simulink model "final_2017"  (R2017b)
settings: Solver=FixedStepAuto  StartTime=0.0  StopTime=inf  FixedStep=0.01  RelTol=1e-3  EnableMultiTasking=on
libraries: arduinolib x12, simulink x3
settings Model: ExtModeTrigDuration=2  Creator=Sina  LastModifiedBy=sina_
settings DataIOCC: ReturnWorkspaceOutputs=on
settings OptimizationCC: EnhancedBackFolding=on  PassReuseOutputArgsAs=Individual arguments  ZeroExternalMemoryAtStartup=off  ZeroInternalMemoryAtStartup=off  MaxStackSize=64  OptimizeBlockOrder=speed  DifferentSizesBufferReuse=on
settings DebuggingCC: ParameterTunabilityLossMsg=error  UnconnectedInputMsg=none  UnconnectedOutputMsg=none  UnconnectedLineMsg=none  SFMachineParentedDataDiag=error
settings HardwareCC: ProdBitPerInt=16  ProdBitPerPointer=16  ProdBitPerSizeT=16  ProdBitPerPtrDiffT=16  ProdLargestAtomicFloat=None  ProdWordSize=8  ProdHWDeviceType=Atmel->AVR
settings SFSimCC: SimUseLocalCustomCode=on  MATLABDynamicMemAlloc=off
settings RTWCC: SystemTargetFile=ert.tlc  HardwareBoard=Arduino Uno  TLCOptions=-aInlineSetEventsForThisBaseRateFcn=TLC_FALSE -aSuppressMultiTaskScheduler=TLC_FALSE -aRateBasedStepFcn=1  TemplateMakefile=ert_default_tmf  RTWUseLocalCustomCode=on  Toolchain=Arduino AVR  BuildConfiguration=Faster Runs
settings CodeAppCC: ForceParamTrailComments=on  IgnoreCustomStorageClasses=off  OperatorAnnotations=on  SimulinkDataObjDesc=on  SFDataObjDesc=on  InsertBlockDesc=on
settings ERTTargetCC: SupportContinuousTime=on  SupportVariableSizeSignals=on  ExtModeTransport=3  ExtModeStaticAlloc=on  ExtModeStaticAllocSize=250  ExtModeMexFile=ext_xcp  ExtModeIntrfLevel=Level2 - Open

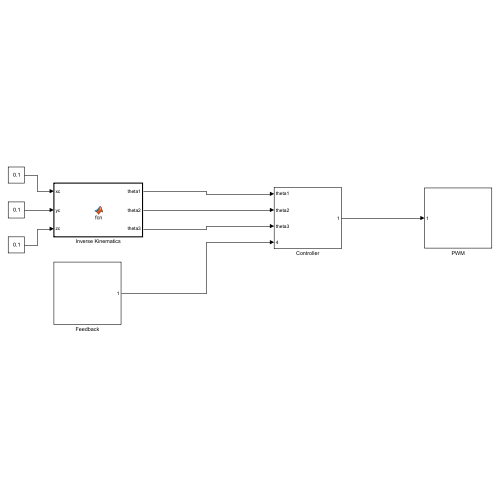
[thumbnail: Simulink's stored preview of the top-level diagram]
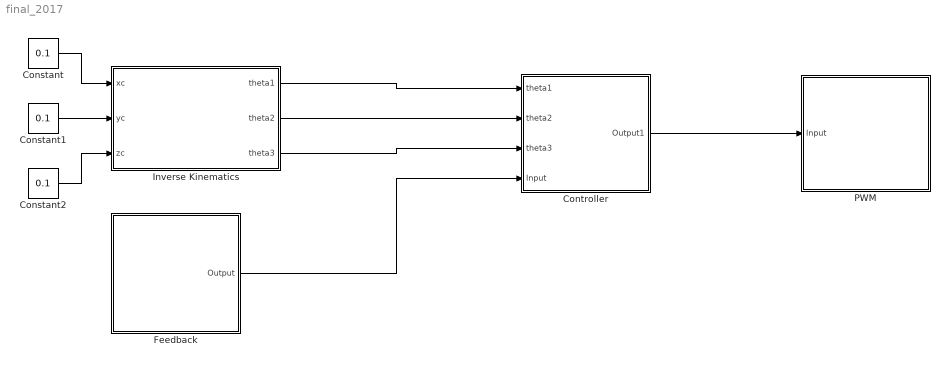
== system final_2017 ==
  Constant : Constant  Value=0.1
  Constant1 : Constant  Value=0.1
  Constant2 : Constant  Value=0.1
  Controller : Subsystem
  Feedback : Subsystem
  Inverse Kinematics : MATLAB Function  TreatAsAtomicUnit=on
  PWM : Subsystem
  wires:
  Feedback/1(Output) -> Controller/4(Input)
  Constant1/1 -> Inverse Kinematics/2(yc)
  Controller/1(Output1) -> PWM/1(Input)
  Constant/1 -> Inverse Kinematics/1(xc)
  Constant2/1 -> Inverse Kinematics/3(zc)
  Inverse Kinematics/1(theta1) -> Controller/1(theta1)
  Inverse Kinematics/2(theta2) -> Controller/2(theta2)
  Inverse Kinematics/3(theta3) -> Controller/3(theta3)

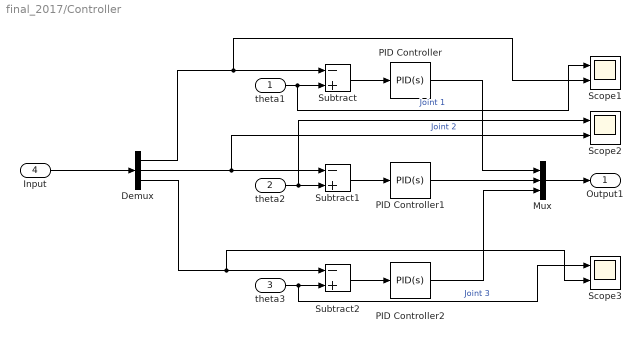
== system final_2017/Controller ==
  theta1 : Inport
  theta2 : Inport  Port=2
  theta3 : Inport  Port=3
  Input : Inport  Port=4
  Demux : Demux  Outputs=3
  Mux : Mux  Inputs=3
  PID Controller : simulink/Continuous/PID Controller  Controller=PID  Form=Parallel  TimeDomain=Continuous-time  SampleTime=-1  IntegratorMethod=Forward Euler  ControllerParametersSource=internal  P=5  I=2  D=1  N=100  UseFilter=on  TunerSelectOption=Transfer Function Based (PID Tuner App)  InitialConditionSource=internal  InitialConditionForIntegrator=0  InitialConditionForFilter=0  DifferentiatorICPrevScaledInput=0  ExternalReset=none  TrackingMode=off  Kt=1  LimitOutput=off  UpperSaturationLimit=inf  LowerSaturationLimit=-inf  LinearizeAsGain=on  AntiWindupMode=none  Kb=1  POutMin=[]  POutMax=[]  IOutMin=[]  IOutMax=[]  DOutMin=[]  DOutMax=[]  NOutMin=[]  NOutMax=[]  SumOutMin=[]  SumOutMax=[]  SaturationOutMin=[]  SaturationOutMax=[]  PParamMin=[]  PParamMax=[]  IParamMin=[]  IParamMax=[]  DParamMin=[]  DParamMax=[]  NParamMin=[]  NParamMax=[]  KbParamMin=[]  KbParamMax=[]  KtParamMin=[]  KtParamMax=[]  KbOutMin=[]  KbOutMax=[]  KtOutMin=[]  KtOutMax=[]  IntegratorOutMin=[]  IntegratorOutMax=[]  FilterOutMin=[]  FilterOutMax=[]  SumI1OutMin=[]  SumI1OutMax=[]  SumI2OutMin=[]  SumI2OutMax=[]  SumI3OutMin=[]  SumI3OutMax=[]  SumDOutMin=[]  SumDOutMax=[]  DifferentiatorOutMin=[]  DifferentiatorOutMax=[]  FilterDiffOutCoefMin=[]  FilterDiffOutCoefMax=[]  ReciprocalOutMin=[]  ReciprocalOutMax=[]  SumDenOutMin=[]  SumDenOutMax=[]  SumNumOutMin=[]  SumNumOutMax=[]  DivideOutMin=[]  DivideOutMax=[]  IntegratorContinuousStateAttributes=''  IntegratorStateMustResolveToSignalObject=off  IntegratorRTWStateStorageClass=Auto  FilterContinuousStateAttributes=''  FilterStateMustResolveToSignalObject=off  FilterRTWStateStorageClass=Auto  InitialConditionSetting=State (most efficient)
  PID Controller1 : simulink/Continuous/PID Controller  Controller=PID  Form=Parallel  TimeDomain=Continuous-time  SampleTime=-1  IntegratorMethod=Forward Euler  ControllerParametersSource=internal  P=5  I=2  D=1  N=100  UseFilter=on  TunerSelectOption=Transfer Function Based (PID Tuner App)  InitialConditionSource=internal  InitialConditionForIntegrator=0  InitialConditionForFilter=0  DifferentiatorICPrevScaledInput=0  ExternalReset=none  TrackingMode=off  Kt=1  LimitOutput=off  UpperSaturationLimit=inf  LowerSaturationLimit=-inf  LinearizeAsGain=on  AntiWindupMode=none  Kb=1  POutMin=[]  POutMax=[]  IOutMin=[]  IOutMax=[]  DOutMin=[]  DOutMax=[]  NOutMin=[]  NOutMax=[]  SumOutMin=[]  SumOutMax=[]  SaturationOutMin=[]  SaturationOutMax=[]  PParamMin=[]  PParamMax=[]  IParamMin=[]  IParamMax=[]  DParamMin=[]  DParamMax=[]  NParamMin=[]  NParamMax=[]  KbParamMin=[]  KbParamMax=[]  KtParamMin=[]  KtParamMax=[]  KbOutMin=[]  KbOutMax=[]  KtOutMin=[]  KtOutMax=[]  IntegratorOutMin=[]  IntegratorOutMax=[]  FilterOutMin=[]  FilterOutMax=[]  SumI1OutMin=[]  SumI1OutMax=[]  SumI2OutMin=[]  SumI2OutMax=[]  SumI3OutMin=[]  SumI3OutMax=[]  SumDOutMin=[]  SumDOutMax=[]  DifferentiatorOutMin=[]  DifferentiatorOutMax=[]  FilterDiffOutCoefMin=[]  FilterDiffOutCoefMax=[]  ReciprocalOutMin=[]  ReciprocalOutMax=[]  SumDenOutMin=[]  SumDenOutMax=[]  SumNumOutMin=[]  SumNumOutMax=[]  DivideOutMin=[]  DivideOutMax=[]  IntegratorContinuousStateAttributes=''  IntegratorStateMustResolveToSignalObject=off  IntegratorRTWStateStorageClass=Auto  FilterContinuousStateAttributes=''  FilterStateMustResolveToSignalObject=off  FilterRTWStateStorageClass=Auto  InitialConditionSetting=State (most efficient)
  PID Controller2 : simulink/Continuous/PID Controller  Controller=PID  Form=Parallel  TimeDomain=Continuous-time  SampleTime=-1  IntegratorMethod=Forward Euler  ControllerParametersSource=internal  P=5  I=2  D=1  N=100  UseFilter=on  TunerSelectOption=Transfer Function Based (PID Tuner App)  InitialConditionSource=internal  InitialConditionForIntegrator=0  InitialConditionForFilter=0  DifferentiatorICPrevScaledInput=0  ExternalReset=none  TrackingMode=off  Kt=1  LimitOutput=off  UpperSaturationLimit=inf  LowerSaturationLimit=-inf  LinearizeAsGain=on  AntiWindupMode=none  Kb=1  POutMin=[]  POutMax=[]  IOutMin=[]  IOutMax=[]  DOutMin=[]  DOutMax=[]  NOutMin=[]  NOutMax=[]  SumOutMin=[]  SumOutMax=[]  SaturationOutMin=[]  SaturationOutMax=[]  PParamMin=[]  PParamMax=[]  IParamMin=[]  IParamMax=[]  DParamMin=[]  DParamMax=[]  NParamMin=[]  NParamMax=[]  KbParamMin=[]  KbParamMax=[]  KtParamMin=[]  KtParamMax=[]  KbOutMin=[]  KbOutMax=[]  KtOutMin=[]  KtOutMax=[]  IntegratorOutMin=[]  IntegratorOutMax=[]  FilterOutMin=[]  FilterOutMax=[]  SumI1OutMin=[]  SumI1OutMax=[]  SumI2OutMin=[]  SumI2OutMax=[]  SumI3OutMin=[]  SumI3OutMax=[]  SumDOutMin=[]  SumDOutMax=[]  DifferentiatorOutMin=[]  DifferentiatorOutMax=[]  FilterDiffOutCoefMin=[]  FilterDiffOutCoefMax=[]  ReciprocalOutMin=[]  ReciprocalOutMax=[]  SumDenOutMin=[]  SumDenOutMax=[]  SumNumOutMin=[]  SumNumOutMax=[]  DivideOutMin=[]  DivideOutMax=[]  IntegratorContinuousStateAttributes=''  IntegratorStateMustResolveToSignalObject=off  IntegratorRTWStateStorageClass=Auto  FilterContinuousStateAttributes=''  FilterStateMustResolveToSignalObject=off  FilterRTWStateStorageClass=Auto  InitialConditionSetting=State (most efficient)
  Scope1 : Scope  NumInputPorts=2
  Scope2 : Scope  NumInputPorts=2
  Scope3 : Scope  NumInputPorts=2
  Subtract : Sum  Inputs=-+
  Subtract1 : Sum  Inputs=-+
  Subtract2 : Sum  Inputs=-+
  Output1 : Outport
  wires:
  PID Controller2/1 -> Mux/3
  Subtract/1 -> PID Controller/1
  Subtract1/1 -> PID Controller1/1
  Subtract2/1 -> PID Controller2/1
  PID Controller/1 -> Mux/1
  PID Controller1/1 -> Mux/2
  theta1/1 -> Scope1/1, Subtract/2  "Joint 1"
  theta2/1 -> Scope2/1, Subtract1/2  "Joint 2"
  theta3/1 -> Scope3/1, Subtract2/2  "Joint 3"
  Input/1 -> Demux/1
  Demux/1 -> Scope1/2, Subtract/1
  Demux/2 -> Scope2/2, Subtract1/1
  Demux/3 -> Scope3/2, Subtract2/1
  Mux/1 -> Output1/1

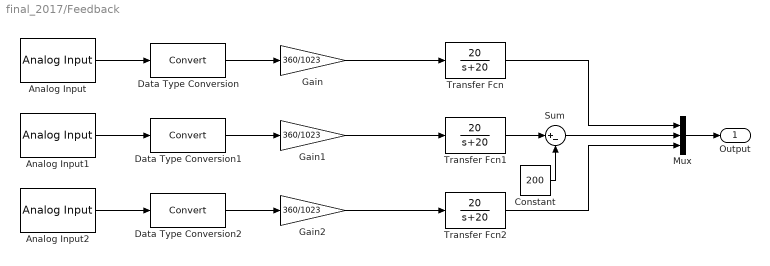
== system final_2017/Feedback ==
  Analog Input : arduinolib/Analog Input  pinNumber=1  ReadResultsOnly=off  ConversionTriggerSource=Software  ExternalTriggerType=uint32( 0 )  OutputDataType=uint16  EnableConversionCompleteNotify=off  EnableOuputStatus=off  SampleTime=0.01  blockPlatform=arduino
  Analog Input1 : arduinolib/Analog Input  pinNumber=2  ReadResultsOnly=off  ConversionTriggerSource=Software  ExternalTriggerType=uint32( 0 )  OutputDataType=uint16  EnableConversionCompleteNotify=off  EnableOuputStatus=off  SampleTime=0.01  blockPlatform=arduino
  Analog Input2 : arduinolib/Analog Input  pinNumber=3  ReadResultsOnly=off  ConversionTriggerSource=Software  ExternalTriggerType=uint32( 0 )  OutputDataType=uint16  EnableConversionCompleteNotify=off  EnableOuputStatus=off  SampleTime=0.01  blockPlatform=arduino
  Constant : Constant  Value=200
  Data Type Conversion : DataTypeConversion
  Data Type Conversion1 : DataTypeConversion
  Data Type Conversion2 : DataTypeConversion
  Gain : Gain  Gain=360/1023
  Gain1 : Gain  Gain=360/1023
  Gain2 : Gain  Gain=360/1023
  Mux : Mux  Inputs=3
  Sum : Sum  Inputs=|+-
  Transfer Fcn : TransferFcn  Numerator=[20]  Denominator=[1 20]
  Transfer Fcn1 : TransferFcn  Numerator=[20]  Denominator=[1 20]
  Transfer Fcn2 : TransferFcn  Numerator=[20]  Denominator=[1 20]
  Output : Outport
  wires:
  Analog Input/1 -> Data Type Conversion/1
  Data Type Conversion/1 -> Gain/1
  Transfer Fcn/1 -> Mux/1
  Gain/1 -> Transfer Fcn/1
  Sum/1 -> Mux/2
  Data Type Conversion1/1 -> Gain1/1
  Analog Input1/1 -> Data Type Conversion1/1
  Analog Input2/1 -> Data Type Conversion2/1
  Data Type Conversion2/1 -> Gain2/1
  Transfer Fcn2/1 -> Mux/3
  Gain2/1 -> Transfer Fcn2/1
  Mux/1 -> Output/1
  Constant/1 -> Sum/2
  Gain1/1 -> Transfer Fcn1/1
  Transfer Fcn1/1 -> Sum/1

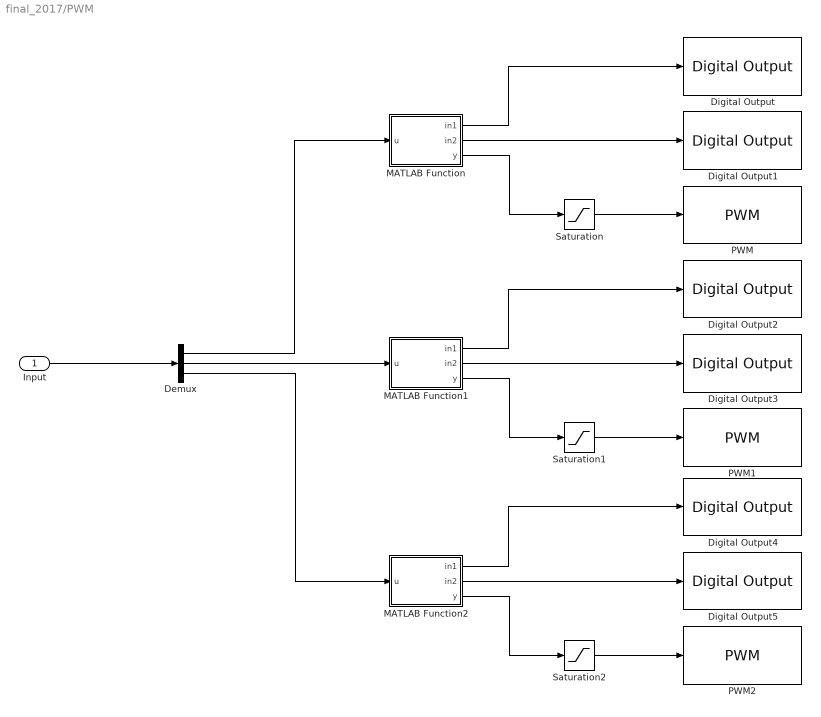
== system final_2017/PWM ==
  Input : Inport
  Demux : Demux  Outputs=3
  Digital Output : arduinolib/Digital Output  pinNumber=12  Direction=output  blockPlatform=arduino
  Digital Output1 : arduinolib/Digital Output  pinNumber=13  Direction=output  blockPlatform=arduino
  Digital Output2 : arduinolib/Digital Output  pinNumber=7  Direction=output  blockPlatform=arduino
  Digital Output3 : arduinolib/Digital Output  pinNumber=8  Direction=output  blockPlatform=arduino
  Digital Output4 : arduinolib/Digital Output  pinNumber=2  Direction=output  blockPlatform=arduino
  Digital Output5 : arduinolib/Digital Output  pinNumber=4  Direction=output  blockPlatform=arduino
  MATLAB Function : MATLAB Function  TreatAsAtomicUnit=on
  MATLAB Function1 : MATLAB Function  TreatAsAtomicUnit=on
  MATLAB Function2 : MATLAB Function  TreatAsAtomicUnit=on
  PWM : arduinolib/PWM  pinNumber=11  frequencyType=Default  desiredFrequency=490.2  achievableFrequency=490.2
  PWM1 : arduinolib/PWM  pinNumber=6  frequencyType=Default  desiredFrequency=490.2  achievableFrequency=490.2
  PWM2 : arduinolib/PWM  pinNumber=5  frequencyType=Default  desiredFrequency=490.2  achievableFrequency=490.2
  Saturation : Saturate  UpperLimit=170  LowerLimit=0
  Saturation1 : Saturate  UpperLimit=170  LowerLimit=0
  Saturation2 : Saturate  UpperLimit=170  LowerLimit=0
  wires:
  MATLAB Function/3(y) -> Saturation/1
  MATLAB Function/2(in2) -> Digital Output1/1
  MATLAB Function/1(in1) -> Digital Output/1
  Saturation/1 -> PWM/1
  Saturation1/1 -> PWM1/1
  MATLAB Function1/1(in1) -> Digital Output2/1
  MATLAB Function1/2(in2) -> Digital Output3/1
  MATLAB Function1/3(y) -> Saturation1/1
  MATLAB Function2/3(y) -> Saturation2/1
  MATLAB Function2/2(in2) -> Digital Output5/1
  MATLAB Function2/1(in1) -> Digital Output4/1
  Saturation2/1 -> PWM2/1
  Demux/1 -> MATLAB Function/1(u)
  Input/1 -> Demux/1
  Demux/2 -> MATLAB Function1/1(u)
  Demux/3 -> MATLAB Function2/1(u)

== matlab function final_2017/PWM/MATLAB Function1 ==
  data: in1 output; in2 output; u input; y output
function [in1,in2,y] = fcn(u)
if u > 0
    in1 = 1;
    in2 = 0;
    y=u;
else
    in1 = 0;
    in2 = 1;
    y = -u;
end

end

== matlab function final_2017/PWM/MATLAB Function ==
  data: in1 output; in2 output; u input; y output
function [in1,in2,y] = fcn(u)
if u > 0
    in1 = 1;
    in2 = 0;
    y=u;
else
    in1 = 0;
    in2 = 1;
    y = -u;
end

end

== matlab function final_2017/PWM/MATLAB Function2 ==
  data: in1 output; in2 output; u input; y output
function [in1,in2,y] = fcn(u)
if u > 0
    in1 = 1;
    in2 = 0;
    y=u;
else
    in1 = 0;
    in2 = 1;
    y = -u;
end

end

== matlab function final_2017/Inverse Kinematics ==
  data: xc input; theta1 output; yc input; zc input; theta2 output; theta3 output
function [theta1,theta2,theta3] = fcn(xc,yc,zc)
r=sqrt(xc^2+yc^2);
k=0;
a=0.146875;
b=0.03125;
theta1=atan2(xc,yc)*180/pi;
theta3=acos((xc^2+yc^2+(zc-k)^2-a^2-b^2)/(2*a*b))*180/pi;
theta2_mx=zeros(4);
theta2_mx(1)=atan((a*b*sin(theta3)+b^2/2*sin(2*theta3)+r*(zc-k))/(r^2-a^2-b^2*(cos(theta3))^2-2*a*b*cos(theta3)));
theta2_mx(2)=theta2_mx(1)+pi;
theta2_mx(3)=atan((a*b*sin(theta3)+b^2/2*sin(2*theta3)-r*(zc-k))/(r^2-a^2-b^2*(cos(theta3))^2-2*a*b*cos(theta3)));
theta2_mx(4)=theta2_mx(3)+pi;
x=a*cos(theta1)*sin(theta2_mx)+b*cos(theta1)*sin(theta2_mx+theta3);
y=a*sin(theta1)*sin(theta2_mx)+b*sin(theta1)*sin(theta2_mx+theta3);
z=k+a*cos(theta2_mx)+b*cos(theta2_mx+theta3);
theta2=0;
for i=1:4;
    if abs(x(i)-xc)<0.001 & abs(y(i)-yc)<0.001 & abs(z(i)-zc)<0.001
        theta2=theta2_mx(i)*180/pi;
        break;
    end
end
theta2=theta2+165;
